simulink model "tut01"  (R2025a)
settings: Solver=VariableStepAuto  StartTime=0.0  StopTime=10.0  RelTol=1e-3
libraries: NSA_DEVS_SINKS x3, NSA_DEVS_SOURCES x2, NSA_DEVS_MATH_OPERATIONS x1
settings Model: Creator=testi  LastModifiedBy=peter

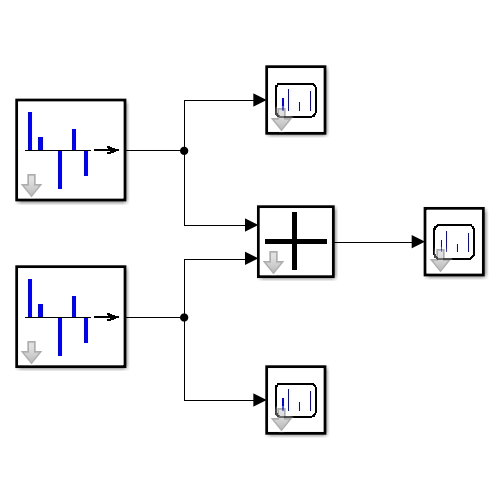
[thumbnail: Simulink's stored preview of the top-level diagram]
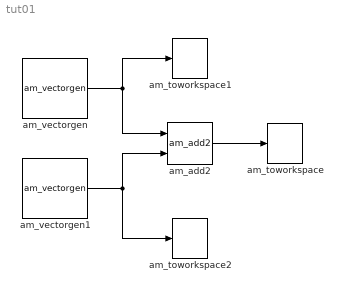
== system tut01 ==
  am_add2 : NSA_DEVS_MATH_OPERATIONS/am_add2  tau=[0,1]  debug=0
      settings: SourceProductName=Math Operations
  am_toworkspace : NSA_DEVS_SINKS/am_toworkspace  varname="\"out1\""  t0=0  format="\"vector\""  tau=[0,5]  debug=0
      settings: SourceProductName=Sinks
  am_toworkspace1 : NSA_DEVS_SINKS/am_toworkspace  varname="\"in1\""  t0=0  format="\"vector\""  tau=[0,5]  debug=0
      settings: SourceProductName=Sinks
  am_toworkspace2 : NSA_DEVS_SINKS/am_toworkspace  varname="\"in2\""  t0=0  format="\"vector\""  tau=[0,5]  debug=0
      settings: SourceProductName=Sinks
  am_vectorgen : NSA_DEVS_SOURCES/am_vectorgen  tvec=[1, 2, 3, 4, 5 ]  yvec=[1, 2, 3, 2, 1]  tau=[0,1]  debug=0
      settings: SourceProductName=Sources
  am_vectorgen1 : NSA_DEVS_SOURCES/am_vectorgen  tvec="[1.3,  2.3, 3, 4, 4.6]"  yvec=[1, 2, 1, 3, 1]  tau=[0,1]  debug=0
      settings: SourceProductName=Sources
  wires:
  am_vectorgen/1 -> am_toworkspace1/1, am_add2/1
  am_vectorgen1/1 -> am_add2/2, am_toworkspace2/1
  am_add2/1 -> am_toworkspace/1
